simulink model "BLOCK_DIAGRAM1"  (R2023b)
settings: Solver=VariableStepAuto  StartTime=0.0  StopTime=10.0  RelTol=1e-3
undefined symbols (not defined in the file): G1_den, G1_num, G2_den, G2_num, G3_den, H1_den, H1_num, H2_den, H2_num, H3_den, H3_num, Tf_den_final, Tf_num_final
settings Model: Creator=Patrick James  LastModifiedBy=Patrick James

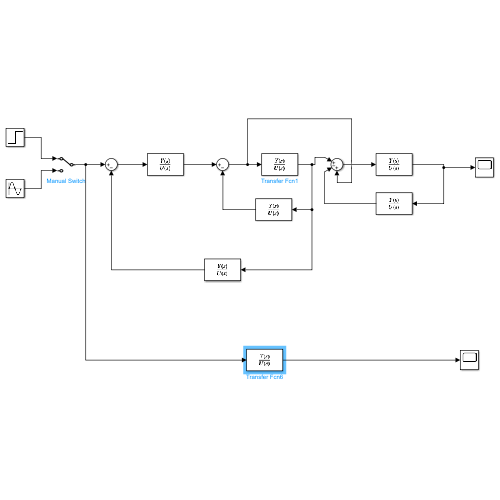
[thumbnail: Simulink's stored preview of the top-level diagram]
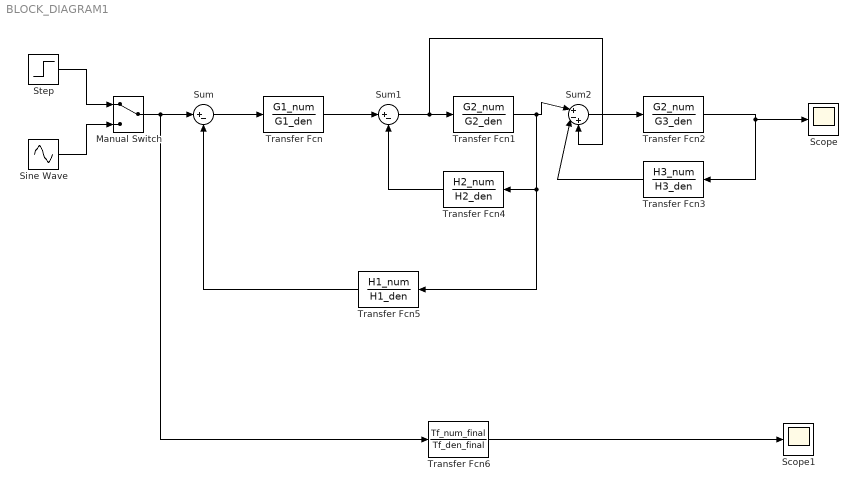
== system BLOCK_DIAGRAM1 ==
  Manual Switch : ManualSwitch
  Scope : Scope
  Scope1 : Scope
  Sine Wave : Sin  SampleTime=0
  Step : Step  SampleTime=0
  Sum : Sum  Inputs=|+-
  Sum1 : Sum  Inputs=|+-
  Sum2 : Sum  Inputs=|+-+
  Transfer Fcn : TransferFcn  Numerator=G1_num  Denominator=G1_den
  Transfer Fcn1 : TransferFcn  Numerator=G2_num  Denominator=G2_den
  Transfer Fcn2 : TransferFcn  Numerator=G2_num  Denominator=G3_den
  Transfer Fcn3 : TransferFcn  Numerator=H3_num  Denominator=H3_den
  Transfer Fcn4 : TransferFcn  Numerator=H2_num  Denominator=H2_den
  Transfer Fcn5 : TransferFcn  Numerator=H1_num  Denominator=H1_den
  Transfer Fcn6 : TransferFcn  Numerator=Tf_num_final  Denominator=Tf_den_final
  wires:
  Step/1 -> Manual Switch/1
  Sine Wave/1 -> Manual Switch/2
  Manual Switch/1 -> Transfer Fcn6/1, Sum/1
  Sum/1 -> Transfer Fcn/1
  Transfer Fcn/1 -> Sum1/1
  Sum1/1 -> Sum2/3, Transfer Fcn1/1
  Transfer Fcn1/1 -> Transfer Fcn5/1, Transfer Fcn4/1, Sum2/1
  Sum2/1 -> Transfer Fcn2/1
  Transfer Fcn2/1 -> Scope/1, Transfer Fcn3/1
  Transfer Fcn3/1 -> Sum2/2
  Transfer Fcn4/1 -> Sum1/2
  Transfer Fcn5/1 -> Sum/2
  Transfer Fcn6/1 -> Scope1/1
